simulink model "bai1_PD_trained_cach2"  (R2017b)
settings: Solver=ode5  StartTime=0.0  StopTime=60  FixedStep=0.01  RelTol=1e-3
undefined symbols (not defined in the file or in its folder): sigbuilder_block
libraries: neural x505
(part 4 of 4)

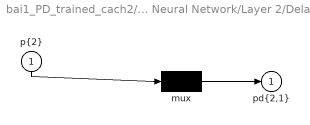
== system bai1_PD_trained_cach2/Custom Neural Network/Layer 2/Delays 1 ==
  "p{2}" : Inport  PortDimensions=500
      mask Display: e = 0.06;c1 = [120 230 180]/255;c2 = ([120 230 180]+0)/(256+128);c3 = ([120 230 180]+128)/(256+128);patch([0 1 1 0],[0 0 1 1],c1);patch([0 1 1 1-e 1-e 0+e],[0 0 1 1-e 0+e 0+e],c2);patch([0 0 1 1-e 0+e 0+e],[0 1 1 1-e 1-e 0+e],c3);plot([0 1 1 0 0],[0 0 1 1 0]);
  mux : Mux  Inputs=1
      mask Display: e = 0.06;c1 = [120 150 230]/255;c2 = ([120 150 230]+0)/383;c3 = ([120 150 230]+128)/383;patch([0 1 1 0],[0 0 1 1],c1);patch([0 1 1 1-e 1-e 0+e],[0 0 1 1-e 0+e 0+e],c2);patch([0 0 1 1-e 0+e 0+e],[0 1 1 1-e 1-e 0+e],c3);plot([0 1 1 0 0],[0 0 1 1 0]);disp('Mux')
  "pd{2,1}" : Outport
      mask Display: e = 0.06;c1 = [120 230 180]/255;c2 = ([120 230 180]+0)/(256+128);c3 = ([120 230 180]+128)/(256+128);patch([0 1 1 0],[0 0 1 1],c1);patch([0 1 1 1-e 1-e 0+e],[0 0 1 1-e 0+e 0+e],c2);patch([0 0 1 1-e 0+e 0+e],[0 1 1 1-e 1-e 0+e],c3);plot([0 1 1 0 0],[0 0 1 1 0]);
  wires:
  "p{2}"/1 -> mux/1
  mux/1 -> "pd{2,1}"/1

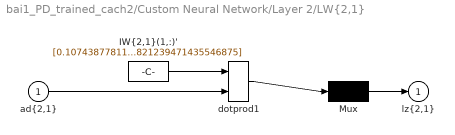
== system bai1_PD_trained_cach2/Custom Neural Network/Layer 2/LW{2,1} ==
  "ad{2,1}" : Inport  PortDimensions=500
      mask Display: e = 0.06;c1 = [120 230 180]/255;c2 = ([120 230 180]+0)/(256+128);c3 = ([120 230 180]+128)/(256+128);patch([0 1 1 0],[0 0 1 1],c1);patch([0 1 1 1-e 1-e 0+e],[0 0 1 1-e 0+e 0+e],c2);patch([0 0 1 1-e 0+e 0+e],[0 1 1 1-e 1-e 0+e],c3);plot([0 1 1 0 0],[0 0 1 1 0]);
  "IW{2,1}(1,:)'" : Constant  Value=[0.10743877811032910563060482900255010463297367095947265625;-0.4136485393802551424613511699135415256023406982421875;1.041351345016968910073273946181870996952056884765625;-0.60330684240151366548587930083158425986766815185546875;0.257558413158241628071465356697444804012775421142578125;0.184898798595594826554844303245772607624530792236328125;-0.1781654064605343312788221510345465503633022308349609375;-0.83429824319338241611632156491396017372608184814453125;-0.7349036640158257416288734020781703293323516845703125;0.004355175634786359085970364191098269657231867313385009765625;-0.5021612301363749253368951031006872653961181640625;0.51508207085225310439824397690244950354099273681640625;-0.433962200606425374527219673836953006684780120849609375;0.94955283426841419203157101946999318897724151611328125;0.29531482560792643443647875756141729652881622314453125;0.1893955089413767722827941497598658315837383270263671875;-0.461504581377388534146888332543312571942806243896484375;0.86731808165561086187977934969239868223667144775390625;-0.5166997954574938933802741303225047886371612548828125;0.80164792044680732718830995509051717817783355712890625;-0.657074030029914712969230095040984451770782470703125;-0.10978118630609391692676268803552375175058841705322265625;-0.96288377293239968413018914361600764095783233642578125;0.185647533853653678992401410141610540449619293212890625;-0.724377590281095162794144926010631024837493896484375;-0.9762528381948849531823952929698862135410308837890625;0.299660383538224939226068954667425714433193206787109375;-0.257630630152472284155606985223130322992801666259765625;0.273889918057194148293120861126226373016834259033203125;-0.079506135846048098247962343521066941320896148681640625;0.0704319742023135908493003398689324967563152313232421875;-0.77300072070732450679741987187298946082592010498046875;0.56615455674796655305414105896488763391971588134765625;0.54674117754383166900566948243067599833011627197265625;0.55627751455020391091466080979444086551666259765625;0.53211651098092416223295231247902847826480865478515625;-0.3718934215238822726945500107831321656703948974609375;0.298401714835268450087824021466076374053955078125;0.0188707699875049449145247848491635522805154323577880859375;0.16907101826828985213779787954990752041339874267578125;-0.34625742817163451814366226244601421058177947998046875;-0.352782763249506248204312441885122098028659820556640625;-0.2475042508320703660285033720356295816600322723388671875;-0.6768312931788920128184372515534050762653350830078125;0.296985323382249422063949850780772976577281951904296875;0.63459825918305179381917469072504900395870208740234375;-0.8730291022875906747913177241571247577667236328125;-0.067496531310243856882635782312718220055103302001953125;-0.585534861108219839564981157309375703334808349609375;0.465369272198674688301167634563171304762363433837890625;1.0618580020818051412589966275845654308795928955078125;-1.0049199593206168401593458838760852813720703125;1.0433951267425352060769228046410717070102691650390625;-0.824830234212119872694302102900110185146331787109375;0.371211864222430631965465863686404190957546234130859375;0.74523102485368364344964220435940660536289215087890625;-0.07053189987841591845896260792869725264608860015869140625;0.50096818416828636788551420977455563843250274658203125;0.750655962210790672628490938222967088222503662109375;-0.00819585746222130893945401197697719908319413661956787109375;-0.46654690102185736311213304361444897949695587158203125;-0.46945581686638726548466138410731218755245208740234375;-0.77605230312348061350036232397542335093021392822265625;-1.055187169860560825185302746831439435482025146484375;-0.66542097611596695561075875957612879574298858642578125;0.5875257655120000865878182594315148890018463134765625;0.75212140496581714188550904509611427783966064453125;-0.15226376213193038022808423193055205047130584716796875;-0.3857637997035732180250988676561973989009857177734375;1.0151399893865413748272885641199536621570587158203125 ...(+24371 chars)]
      mask Display: e = 0.06;c1 = [120 150 230]/255;c2 = ([120 150 230]+0)/383;c3 = ([120 150 230]+128)/383;patch([0 1 1 0],[0 0 1 1],c1);patch([0 1 1 1-e 1-e 0+e],[0 0 1 1-e 0+e 0+e],c2);patch([0 0 1 1-e 0+e 0+e],[0 1 1 1-e 1-e 0+e],c3);plot([0 1 1 0 0],[0 0 1 1 0]);disp('weights');
  Mux : Mux  Inputs=1
      mask Display: e = 0.06;c1 = [120 150 230]/255;c2 = ([120 150 230]+0)/383;c3 = ([120 150 230]+128)/383;patch([0 1 1 0],[0 0 1 1],c1);patch([0 1 1 1-e 1-e 0+e],[0 0 1 1-e 0+e 0+e],c2);patch([0 0 1 1-e 0+e 0+e],[0 1 1 1-e 1-e 0+e],c3);plot([0 1 1 0 0],[0 0 1 1 0]);disp('Mux');
  dotprod1 : neural/Weight Functions/dotprod
  "lz{2,1}" : Outport
      mask Display: e = 0.06;c1 = [120 230 180]/255;c2 = ([120 230 180]+0)/(256+128);c3 = ([120 230 180]+128)/(256+128);patch([0 1 1 0],[0 0 1 1],c1);patch([0 1 1 1-e 1-e 0+e],[0 0 1 1-e 0+e 0+e],c2);patch([0 0 1 1-e 0+e 0+e],[0 1 1 1-e 1-e 0+e],c3);plot([0 1 1 0 0],[0 0 1 1 0]);
  wires:
  "IW{2,1}(1,:)'"/1 -> dotprod1/1
  "ad{2,1}"/1 -> dotprod1/2
  dotprod1/1 -> Mux/1
  Mux/1 -> "lz{2,1}"/1
